simulink model "lvpp2d"  (Simulink 3.00)
settings: Solver=ode45  SolverMode=SingleTasking  StartTime=0.0  StopTime=20  RelTol=1e-3  AbsTol=1e-6
undefined symbols (not defined in the file or in its folder): sfunxyz
settings Model: ExternalInput=[]  SaveTime=off  SaveOutput=off  InitialState=[]  IntegerOverflowMsg=none  RTWOptions="-aEnforceIntegerDowncast=1 -aFoldNonRolledExpr=1 -aInlineInvariantSignals=1 -aInlineParameters=0 -aLocalBlockOutputs=1 -aRollThreshold=5 -aZeroInternalMemoryAtStartup=1 -aZeroExternalMemoryAtStartup=1 -aInitFltsAndDblsToZero=1 -aGenerateReport=0 -aGenCodeOnly=0 -aRTWVerbose=1 -aIncludeHyperlinkInReport=0 -aLaunchReport=0 -aForceParamTrailComments=0 -aGenerateComments=1 -aIgnoreCustomStorageClasses=1 -aIncHierarchyInIds=0 -aMaxRTWIdLen=31 -aShowEliminatedStatements=0 -aPrefixModelToSubsysFcnNames=1 -aIncDataTypeInIds=0 -aInsertBlockDesc=0 -aSimulinkBlockComments=1 -aInlinedPrmAccess=\"Literals\"  -aSuppressErrorStatus=0 -aModelReferenceCompliant=1 -aSupportNonInlinedSFcns=1 -aSupportContinuousTime=1 -aSupportComplex=1 -aSupportNonFinite=1 -aSupportAbsoluteTime=1 -aTargetFcnLib=\"ansi_tfl_tmw.mat\" -aMultiInstanceERTCode=0 -aLogVarNameModifier=\"rt_\" -aIsPILTarget=0 -aCombineOutputUpdateFcns=0 -aGenerateASAP2=0 -aGenerateSampleERTMain=0 -aGenerateFullHeader=1 -aUtilityFuncGeneration=\"Auto\" -aIncludeFileDelimiter=\"Auto\" -aIncludeMdlTerminateFcn=1 -aPurelyIntegerCode=0 -aERTCustomFileBanners=0 -aRTWCAPIStates=0 -aRTWCAPIParams=0 -aRTWCAPISignals=0 -aMatFileLogging=1 -aGenFloatMathFcnCalls=\"ANSI_C\" -aExtModeMexFile=\"ext_comm\" -aExtModeTransport=0 -aExtModeStaticAllocSize=1000000 -aExtModeTesting=0 -aExtModeStaticAlloc=0 -aExtMode=0  -aInitFltsAndDblsToZero=1 -aInitFltsAndDblsToZero=1 -aInitFltsAndDblsToZero=1"  Creator=The MathWorks Inc.  LastModifiedBy=campa

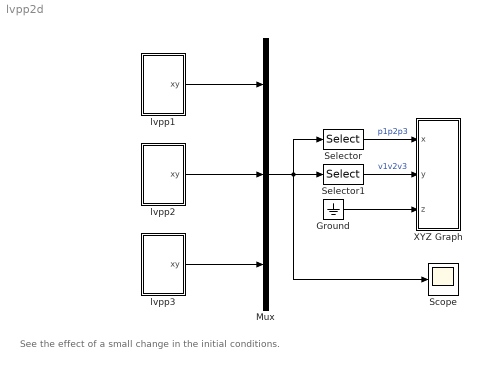
== system lvpp2d ==
  note: See the effect of a small change in the initial conditions.
  Ground : Ground
  Mux : Mux  Inputs=[2 2 2]
  Scope : Scope
      settings: TimeRange=20  YMin=0  YMax=400  SaveToWorkspace=off  SaveName=ScopeData
  Selector : Selector  Elements=[1 3 5]  InputPortWidth=6
  Selector1 : Selector  Elements=[2 4 6]  InputPortWidth=6
  XYZ Graph : Subsystem  LoadFcn=sfunxyz([],[],[],'LoadBlock')  StartFcn=sfunxyz([],[],[],'Start')  StopFcn=sfunxyz([],[],[],'Stop')  mask(XYZ multiscope){np=3, xlim=[-400 400], ylim=[-400 400], zlim=[0 1], cp=[0 0 1], gd=on, st=0.01}
      mask prompts: np "Number of lines"; xlim "[xmin xmax]"; ylim "[ymin ymax]"; zlim "[zmin zmax]"; cp "Camera position (use [0 0 1] for 2D XY view)"; gd "Grid"; st "Sample time:"
      mask help:
      | Multidimensional XYZ scope using MATLAB graph window.
      |    X,Y,Z coordinates are respectively the first,second, and third input.
      |    Enter the number of lines, the XYZ ranges, the camera position,
      |    and the sampling time, as mask parameters.
      settings: CopyFcn=sfunxyz([],[],[],'CopyBlock')  DeleteFcn=sfunxyz([],[],[],'DeleteBlock')  NameChangeFcn=sfunxyz([],[],[],'NameChange')
      mask Help:
      | This block can be used to explore limit cycles.
      |    Look at the m-file sfunxyz.m to see how it works.
      mask Display: plot([.05 .95 .95 .05 .05],[.45 .45 .95 .95 .45], 0.5+cos(0:0.1:2*pi)*0.3,0.7+sin(0:0.1:2*pi)*0.2)
  lvpp1 : Subsystem  mask(Lotka Volterra System){a=1, b=0.01, c=1, d=0.02, xy0=[20 20]}
      mask prompts: xy0 "Initial point p0 = [x0 y0]"
      mask help:
      | This autonomous system represents the lotka volterra prey predator model:
      |  xdot =  ax - bxy;   ydot = -cy +dxy
      |  where x represents the prey and y represents the predator.
      |  Parameters and initial state can be selected from the mask.
      mask Help:
      | This autonomous system represents the lotka volterra prey predator model.
      |  <p>
      |  The system equations are:
      |  xdot =  ax - bxy
      |  ydot = -cy +dxy
      |  where x represents the prey and y represents the predator.
      |  Parameters and initial state can be selected from the mask.
  lvpp2 : Subsystem  mask(Lotka Volterra System){a=1, b=0.01, c=1, d=0.02, xy0=[30 60]}
      mask prompts: xy0 "Initial point p0 = [x0 y0]"
      mask help:
      | This autonomous system represents the lotka volterra prey predator model:
      |  xdot =  ax - bxy;   ydot = -cy +dxy
      |  where x represents the prey and y represents the predator.
      |  Parameters and initial state can be selected from the mask.
      mask Help:
      | This autonomous system represents the lotka volterra prey predator model.
      |  <p>
      |  The system equations are:
      |  xdot =  ax - bxy
      |  ydot = -cy +dxy
      |  where x represents the prey and y represents the predator.
      |  Parameters and initial state can be selected from the mask.
  lvpp3 : Subsystem  mask(Lotka Volterra System){a=1, b=0.01, c=1, d=0.02, xy0=[50 100]*0.9}
      mask prompts: xy0 "Initial point p0 = [x0 y0]"
      mask help:
      | This autonomous system represents the lotka volterra prey predator model:
      |  xdot =  ax - bxy;   ydot = -cy +dxy
      |  where x represents the prey and y represents the predator.
      |  Parameters and initial state can be selected from the mask.
      mask Help:
      | This autonomous system represents the lotka volterra prey predator model.
      |  <p>
      |  The system equations are:
      |  xdot =  ax - bxy
      |  ydot = -cy +dxy
      |  where x represents the prey and y represents the predator.
      |  Parameters and initial state can be selected from the mask.
  wires:
  Mux/1 -> Selector1/1, Selector/1, Scope/1
  Selector/1 -> XYZ Graph/1(x)  "p1p2p3"
  Selector1/1 -> XYZ Graph/2(y)  "v1v2v3"
  Ground/1 -> XYZ Graph/3(z)
  lvpp1/1(xy) -> Mux/1
  lvpp2/1(xy) -> Mux/2
  lvpp3/1(xy) -> Mux/3

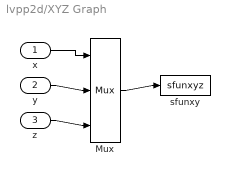
== system lvpp2d/XYZ Graph ==
  x : Inport  Port=1  PortWidth=-1  SampleTime=-1  DataType=auto
      settings: SignalType=auto
  y : Inport  Port=2  PortWidth=-1  SampleTime=-1  DataType=auto
      settings: SignalType=auto
  z : Inport  Port=3  PortWidth=-1  SampleTime=-1  DataType=auto
      settings: SignalType=auto
  Mux : Mux  Inputs=[np np np]
      settings: DisplayOption=none
  sfunxy : S-Function  FunctionName=sfunxyz  Parameters=[xlim ylim zlim],st,np,cp,gd  PortCounts=[]  SFunctionModules=''
  wires:
  z/1 -> Mux/3
  y/1 -> Mux/2
  x/1 -> Mux/1
  Mux/1 -> sfunxy/1

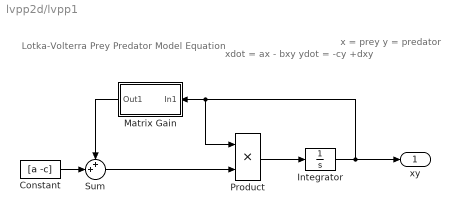
== system lvpp2d/lvpp1 ==
  note: Lotka-Volterra Prey Predator Model Equation
  note: xdot =  ax - bxy
      | ydot = -cy +dxy
  note: x = prey
      | y = predator
  Constant : Constant  Value=[a -c]
  Integrator : Integrator  ExternalReset=none  InitialConditionSource=internal  InitialCondition=xy0  LimitOutput=off  UpperSaturationLimit=inf  LowerSaturationLimit=-inf  ShowSaturationPort=off  ShowStatePort=off  AbsoluteTolerance=auto
  Matrix Gain : Subsystem  Orientation=left  mask(Matrix Gain){K=[0 -b;d 0]}
      mask prompts: K "Gain matrix:"
      mask help: Matrix Gain.
      mask Help: Multiplies input vector by entered matrix to produce output vector (y=Au).
      mask Display: disp('[0 -b; d 0]')
  Product : Product  Inputs=2  SaturateOnIntegerOverflow=on
  Sum : Sum  Inputs=++|  SaturateOnIntegerOverflow=off
  xy : Outport  Port=1
  wires:
  Constant/1 -> Sum/2
  Matrix Gain/1(Out1) -> Sum/1
  Product/1 -> Integrator/1
  Integrator/1 -> xy/1, Product/1, Matrix Gain/1(In1)
  Sum/1 -> Product/2

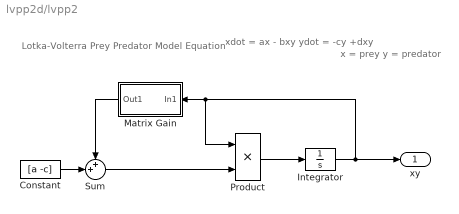
== system lvpp2d/lvpp2 ==
  note: x = prey
      | y = predator
  note: xdot =  ax - bxy
      | ydot = -cy +dxy
  note: Lotka-Volterra Prey Predator Model Equation
  Constant : Constant  Value=[a -c]
  Integrator : Integrator  ExternalReset=none  InitialConditionSource=internal  InitialCondition=xy0  LimitOutput=off  UpperSaturationLimit=inf  LowerSaturationLimit=-inf  ShowSaturationPort=off  ShowStatePort=off  AbsoluteTolerance=auto
  Matrix Gain : Subsystem  Orientation=left  mask(Matrix Gain){K=[0 -b;d 0]}
      mask prompts: K "Gain matrix:"
      mask help: Matrix Gain.
      mask Help: Multiplies input vector by entered matrix to produce output vector (y=Au).
      mask Display: disp('[0 -b; d 0]')
  Product : Product  Inputs=2  SaturateOnIntegerOverflow=on
  Sum : Sum  Inputs=++|  SaturateOnIntegerOverflow=off
  xy : Outport  Port=1
  wires:
  Sum/1 -> Product/2
  Integrator/1 -> Matrix Gain/1(In1), Product/1, xy/1
  Product/1 -> Integrator/1
  Matrix Gain/1(Out1) -> Sum/1
  Constant/1 -> Sum/2

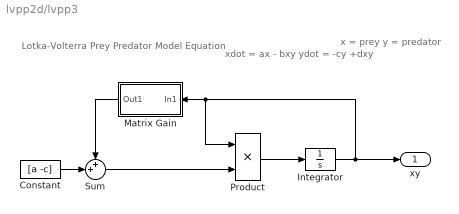
== system lvpp2d/lvpp3 ==
  note: Lotka-Volterra Prey Predator Model Equation
  note: xdot =  ax - bxy
      | ydot = -cy +dxy
  note: x = prey
      | y = predator
  Constant : Constant  Value=[a -c]
  Integrator : Integrator  ExternalReset=none  InitialConditionSource=internal  InitialCondition=xy0  LimitOutput=off  UpperSaturationLimit=inf  LowerSaturationLimit=-inf  ShowSaturationPort=off  ShowStatePort=off  AbsoluteTolerance=auto
  Matrix Gain : Subsystem  Orientation=left  mask(Matrix Gain){K=[0 -b;d 0]}
      mask prompts: K "Gain matrix:"
      mask help: Matrix Gain.
      mask Help: Multiplies input vector by entered matrix to produce output vector (y=Au).
      mask Display: disp('[0 -b; d 0]')
  Product : Product  Inputs=2  SaturateOnIntegerOverflow=on
  Sum : Sum  Inputs=++|  SaturateOnIntegerOverflow=off
  xy : Outport  Port=1
  wires:
  Constant/1 -> Sum/2
  Matrix Gain/1(Out1) -> Sum/1
  Product/1 -> Integrator/1
  Integrator/1 -> xy/1, Product/1, Matrix Gain/1(In1)
  Sum/1 -> Product/2

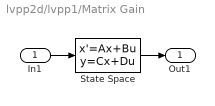
== system lvpp2d/lvpp1/Matrix Gain ==
  In1 : Inport  Port=1  PortWidth=-1  SampleTime=-1  DataType=auto
      settings: SignalType=auto
  State Space : StateSpace  A=[]  B=[]  C=[]  D=K  X0=0
  Out1 : Outport  Port=1
  wires:
  In1/1 -> State Space/1
  State Space/1 -> Out1/1

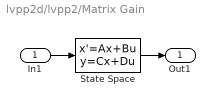
== system lvpp2d/lvpp2/Matrix Gain ==
  In1 : Inport  Port=1  PortWidth=-1  SampleTime=-1  DataType=auto
      settings: SignalType=auto
  State Space : StateSpace  A=[]  B=[]  C=[]  D=K  X0=0
  Out1 : Outport  Port=1
  wires:
  State Space/1 -> Out1/1
  In1/1 -> State Space/1

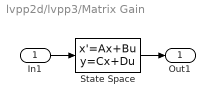
== system lvpp2d/lvpp3/Matrix Gain ==
  In1 : Inport  Port=1  PortWidth=-1  SampleTime=-1  DataType=auto
      settings: SignalType=auto
  State Space : StateSpace  A=[]  B=[]  C=[]  D=K  X0=0
  Out1 : Outport  Port=1
  wires:
  In1/1 -> State Space/1
  State Space/1 -> Out1/1
